simulink library "platooning_custom_blocks"  (R2018b)
settings: Solver=VariableStepAuto  StartTime=0.0  StopTime=10.0  RelTol=1e-3
undefined symbols (not defined in the file): AccPdl_pdlbpt, AccPdl_spdbpt, AccPdl_trqMap, adj_motEffMap, BETModel, BrkPdl_brkTrq, BrkPdl_pdlbpt, Cd_Map, Cd_Map_T2, CT_accPdl_pdlbpt, CT_accPdl_spdbpt, CT_accPdl_trqMap, CT_brkPdl_brkTrq, CT_brkPdl_pdlbpt, CTModel, d_11, d_22, DiscIntNeverNeededParam, init_veh_spd_mps, max_Cd_frac, min_Cd_frac, motSpdVec, motTrqVec, msk_init_pos_m, msk_mot_cont_trq, msk_mot_num, msk_mot_spd_bpt, N_OptResults, sim_t_step, simDrv, SPHETModel, t_step
libraries: simulink x19, $bdroot x16, dspstat3 x2, custom_func x1
(part 2 of 5)

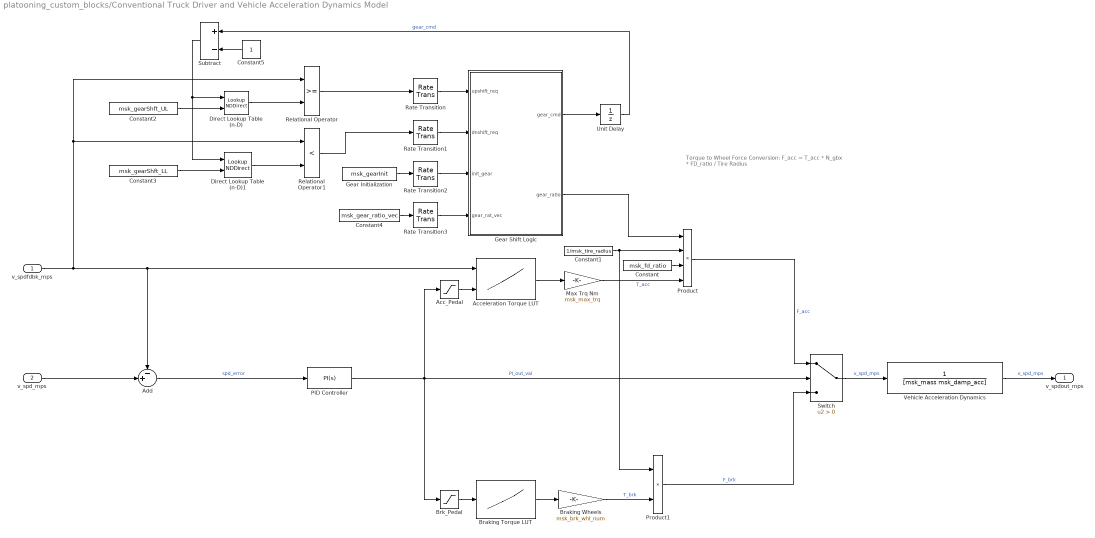
== system platooning_custom_blocks/Conventional Truck Driver and Vehicle Acceleration Dynamics Model ==
  note: Torque to Wheel Force Conversion:
      | F_acc = T_acc * N_gbx * FD_ratio / Tire Radius
  v_spdfdbk_mps : Inport
  v_spd_mps : Inport  Port=2
  Acc_Pedal : Saturate  UpperLimit=1  LowerLimit=0
  Acceleration Torque LUT : Lookup_n-D  BreakpointsForDimension1=msk_acc_spdbpt  BreakpointsForDimension2=msk_acc_pdlbpt  Table=msk_acc_trqmap  InternalRulePriority=Speed  RndMeth=Simplest  InputSameDT=on
  Add : Sum  Inputs=-+|
  Braking Torque LUT : Lookup_n-D  NumberOfTableDimensions=1  BreakpointsForDimension1=msk_brk_pdlbpt  Table=msk_brk_trq  InternalRulePriority=Speed  RndMeth=Simplest  InputSameDT=on
  Braking Wheels : Gain  Gain=msk_brk_whl_num
  Brk_Pedal : Saturate  UpperLimit=0  LowerLimit=-1
  Constant : Constant  Value=msk_fd_ratio
  Constant1 : Constant  Value=1/msk_tire_radius
  Constant2 : Constant  Value=msk_gearShft_UL
  Constant3 : Constant  Value=msk_gearShft_LL
  Constant4 : Constant  Value=msk_gear_ratio_vec
  Constant5 : Constant
  Direct Lookup Table (n-D) : LookupNDDirect  NumberOfTableDimensions=1  TableIsInput=on
  Direct Lookup Table (n-D)1 : LookupNDDirect  NumberOfTableDimensions=1  TableIsInput=on
  Gear Initialization : Constant  Value=msk_gearInit
  Gear Shift Logic : MATLAB Function  TreatAsAtomicUnit=on
  Max Trq Nm : Gain  Gain=msk_max_trq
  PID Controller : simulink/Continuous/PID Controller  Controller=PI  Form=Parallel  TimeDomain=Continuous-time  SampleTime=-1  IntegratorMethod=Forward Euler  FilterMethod=Forward Euler  ControllerParametersSource=internal  P=msk_Kp  I=msk_Ki  D=0  UseFilter=on  N=100  TunerSelectOption=Transfer Function Based (PID Tuner App)  InitialConditionSource=internal  InitialConditionForIntegrator=0  InitialConditionForFilter=0  DifferentiatorICPrevScaledInput=0  ExternalReset=none  TrackingMode=off  Kt=1  LimitOutput=on  UpperSaturationLimit=1  LowerSaturationLimit=-1  LinearizeAsGain=on  AntiWindupMode=clamping  Kb=1  POutMin=[]  POutMax=[]  IOutMin=[]  IOutMax=[]  DOutMin=[]  DOutMax=[]  NOutMin=[]  NOutMax=[]  SumOutMin=[]  SumOutMax=[]  SaturationOutMin=[]  SaturationOutMax=[]  PParamMin=[]  PParamMax=[]  IParamMin=[]  IParamMax=[]  DParamMin=[]  DParamMax=[]  NParamMin=[]  NParamMax=[]  KbParamMin=[]  KbParamMax=[]  KtParamMin=[]  KtParamMax=[]  KbOutMin=[]  KbOutMax=[]  KtOutMin=[]  KtOutMax=[]  IntegratorOutMin=[]  IntegratorOutMax=[]  FilterOutMin=[]  FilterOutMax=[]  SumI1OutMin=[]  SumI1OutMax=[]  SumI2OutMin=[]  SumI2OutMax=[]  SumI3OutMin=[]  SumI3OutMax=[]  SumI4OutMin=[]  SumI4OutMax=[]  SumDOutMin=[]  SumDOutMax=[]  DifferentiatorOutMin=[]  DifferentiatorOutMax=[]  FilterDiffOutCoefMin=[]  FilterDiffOutCoefMax=[]  ReciprocalOutMin=[]  ReciprocalOutMax=[]  SumDenOutMin=[]  SumDenOutMax=[]  SumNumOutMin=[]  SumNumOutMax=[]  DivideOutMin=[]  DivideOutMax=[]  IntegratorContinuousStateAttributes=''  IntegratorStateMustResolveToSignalObject=off  IntegratorRTWStateStorageClass=Auto  FilterContinuousStateAttributes=''  FilterStateMustResolveToSignalObject=off  FilterRTWStateStorageClass=Auto  ParallelPVariant=InternalParameters  IdealPVariant=Disabled  IVariant=InternalParameters  DVariant=Disabled  IntegratorVariant=Continuous  SatVariant=Enabled  AWVariant=ContClampingParallel  PCopyVariant=Disabled  TRVariant=Disabled  FdbkBlocksVariant=Forward  IdealPFdbkVariant=Disabled  SatFdbkVariant=Disabled  DerivativeFilterVariant=Disabled  NVariant=Disabled  NCopyVariant=Disabled_SignalSpec  FilterICVariant=Disabled  IntegratorICVariant=InternalICs  ExternalResetVariant=Disabled  TRSumVariant=Passthrough  SumFdbkVariant=Disabled  SumVariant=Sum_PI
  Product : Product  Inputs=4
  Product1 : Product
  Rate Transition{,1..3} (4 alike) : RateTransition  OutPortSampleTime=msk_t_step
  Relational Operator : RelationalOperator  OutDataTypeStr=boolean  RndMeth=Simplest
  Relational Operator1 : RelationalOperator  Operator=<  OutDataTypeStr=boolean  RndMeth=Simplest
  Subtract : Sum  Inputs=+-
  Switch : Switch  Criteria=u2 > Threshold
  Unit Delay : UnitDelay  SampleTime=-1
  Vehicle Acceleration Dynamics : TransferFcn  Denominator=[msk_mass msk_damp_acc]
  v_spdout_mps : Outport
  wires:
  Switch/1 -> Vehicle Acceleration Dynamics/1  "v_spd_mps"
  Vehicle Acceleration Dynamics/1 -> v_spdout_mps/1  "v_spd_mps"
  Braking Wheels/1 -> Product1/2  "T_brk"
  Max Trq Nm/1 -> Product/4  "T_acc"
  Rate Transition3/1 -> Gear Shift Logic/4(gear_rat_vec)
  Rate Transition2/1 -> Gear Shift Logic/3(init_gear)
  Rate Transition1/1 -> Gear Shift Logic/2(dnshift_req)
  Rate Transition/1 -> Gear Shift Logic/1(upshift_req)
  Braking Torque LUT/1 -> Braking Wheels/1
  PID Controller/1 -> Switch/2, Brk_Pedal/1, Acc_Pedal/1  "PI_out_val"
  Acceleration Torque LUT/1 -> Max Trq Nm/1
  v_spdfdbk_mps/1 -> Relational Operator1/1, Relational Operator/1, Add/1, Acceleration Torque LUT/1
  v_spd_mps/1 -> Add/2
  Product1/1 -> Switch/3  "F_brk"
  Product/1 -> Switch/1  "F_acc"
  Add/1 -> PID Controller/1  "spd_error"
  Acc_Pedal/1 -> Acceleration Torque LUT/2
  Brk_Pedal/1 -> Braking Torque LUT/1
  Constant/1 -> Product/3
  Constant1/1 -> Product1/1, Product/2
  Direct Lookup Table (n-D)/1 -> Relational Operator/2
  Constant2/1 -> Direct Lookup Table (n-D)/2
  Constant3/1 -> Direct Lookup Table (n-D)1/2
  Direct Lookup Table (n-D)1/1 -> Relational Operator1/2
  Relational Operator/1 -> Rate Transition/1
  Relational Operator1/1 -> Rate Transition1/1
  Gear Initialization/1 -> Rate Transition2/1
  Gear Shift Logic/1(gear_cmd) -> Unit Delay/1
  Gear Shift Logic/2(gear_ratio) -> Product/1
  Constant4/1 -> Rate Transition3/1
  Unit Delay/1 -> Subtract/1  "gear_cmd"
  Constant5/1 -> Subtract/2
  Subtract/1 -> Direct Lookup Table (n-D)1/1, Direct Lookup Table (n-D)/1

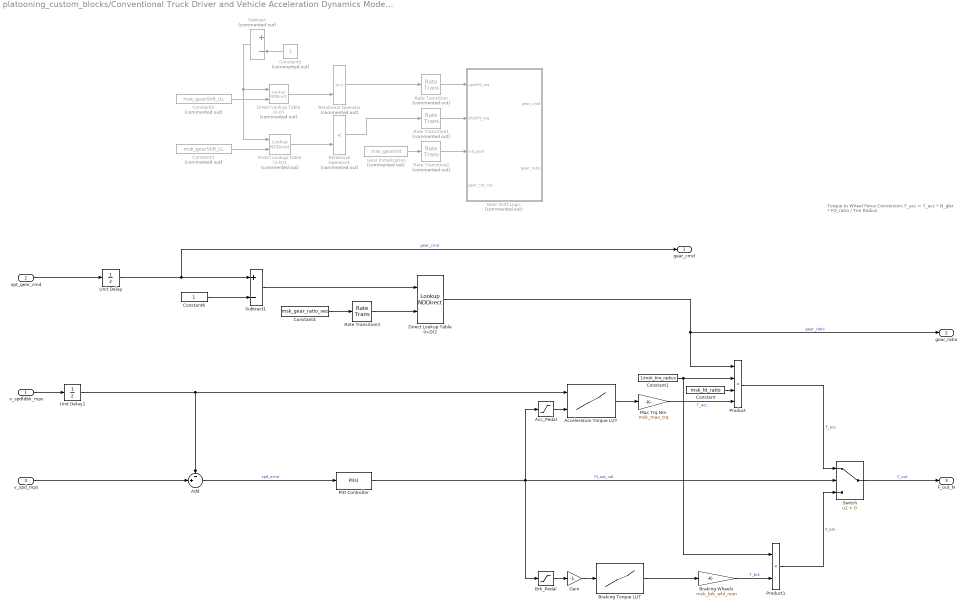
== system platooning_custom_blocks/Conventional Truck Driver and Vehicle Acceleration Dynamics Model - Force Output ==
  note: Torque to Wheel Force Conversion:
      | F_acc = T_acc * N_gbx * FD_ratio / Tire Radius
  v_spdfdbk_mps : Inport
  opt_gear_cmd : Inport  Port=2
  v_spd_mps : Inport  Port=3
  Acc_Pedal : Saturate  UpperLimit=1  LowerLimit=0
  Acceleration Torque LUT : Lookup_n-D  BreakpointsForDimension1=msk_acc_spdbpt  BreakpointsForDimension2=msk_acc_pdlbpt  Table=msk_acc_trqmap  InternalRulePriority=Speed  RndMeth=Simplest  InputSameDT=on
  Add : Sum  Inputs=-+|
  Braking Torque LUT : Lookup_n-D  NumberOfTableDimensions=1  BreakpointsForDimension1=msk_brk_pdlbpt  Table=msk_brk_trq * -1  InternalRulePriority=Speed  RndMeth=Simplest  InputSameDT=on
  Braking Wheels : Gain  Gain=msk_brk_whl_num
  Brk_Pedal : Saturate  UpperLimit=0  LowerLimit=-1
  Constant : Constant  Value=msk_fd_ratio
  Constant1 : Constant  Value=1/msk_tire_radius
  Constant2 : Constant  Commented=on  Value=msk_gearShft_UL
  Constant3 : Constant  Commented=on  Value=msk_gearShft_LL
  Constant4 : Constant  Value=msk_gear_ratio_vec
  Constant5 : Constant  Commented=on
  Constant6 : Constant
  Direct Lookup Table (n-D) : LookupNDDirect  Commented=on  NumberOfTableDimensions=1  TableIsInput=on
  Direct Lookup Table (n-D)1 : LookupNDDirect  Commented=on  NumberOfTableDimensions=1  TableIsInput=on
  Direct Lookup Table (n-D)2 : LookupNDDirect  NumberOfTableDimensions=1  TableIsInput=on
  Gain : Gain  Gain=-1
  Gear Initialization : Constant  Commented=on  Value=msk_gearInit
  Gear Shift Logic : MATLAB Function  Commented=on  TreatAsAtomicUnit=on
  Max Trq Nm : Gain  Gain=msk_max_trq
  PID Controller : simulink/Continuous/PID Controller  Controller=PI  Form=Parallel  TimeDomain=Continuous-time  SampleTime=-1  IntegratorMethod=Forward Euler  FilterMethod=Forward Euler  ControllerParametersSource=internal  P=msk_Kp  I=msk_Ki  D=0  UseFilter=on  N=100  TunerSelectOption=Transfer Function Based (PID Tuner App)  InitialConditionSource=internal  InitialConditionForIntegrator=0  InitialConditionForFilter=0  DifferentiatorICPrevScaledInput=0  ExternalReset=none  TrackingMode=off  Kt=1  LimitOutput=on  UpperSaturationLimit=1  LowerSaturationLimit=-1  LinearizeAsGain=on  AntiWindupMode=clamping  Kb=1  POutMin=[]  POutMax=[]  IOutMin=[]  IOutMax=[]  DOutMin=[]  DOutMax=[]  NOutMin=[]  NOutMax=[]  SumOutMin=[]  SumOutMax=[]  SaturationOutMin=[]  SaturationOutMax=[]  PParamMin=[]  PParamMax=[]  IParamMin=[]  IParamMax=[]  DParamMin=[]  DParamMax=[]  NParamMin=[]  NParamMax=[]  KbParamMin=[]  KbParamMax=[]  KtParamMin=[]  KtParamMax=[]  KbOutMin=[]  KbOutMax=[]  KtOutMin=[]  KtOutMax=[]  IntegratorOutMin=[]  IntegratorOutMax=[]  FilterOutMin=[]  FilterOutMax=[]  SumI1OutMin=[]  SumI1OutMax=[]  SumI2OutMin=[]  SumI2OutMax=[]  SumI3OutMin=[]  SumI3OutMax=[]  SumI4OutMin=[]  SumI4OutMax=[]  SumDOutMin=[]  SumDOutMax=[]  DifferentiatorOutMin=[]  DifferentiatorOutMax=[]  FilterDiffOutCoefMin=[]  FilterDiffOutCoefMax=[]  ReciprocalOutMin=[]  ReciprocalOutMax=[]  SumDenOutMin=[]  SumDenOutMax=[]  SumNumOutMin=[]  SumNumOutMax=[]  DivideOutMin=[]  DivideOutMax=[]  IntegratorContinuousStateAttributes=''  IntegratorStateMustResolveToSignalObject=off  IntegratorRTWStateStorageClass=Auto  FilterContinuousStateAttributes=''  FilterStateMustResolveToSignalObject=off  FilterRTWStateStorageClass=Auto  ParallelPVariant=InternalParameters  IdealPVariant=Disabled  IVariant=InternalParameters  DVariant=Disabled  IntegratorVariant=Continuous  SatVariant=Enabled  AWVariant=ContClampingParallel  PCopyVariant=Disabled  TRVariant=Disabled  FdbkBlocksVariant=Forward  IdealPFdbkVariant=Disabled  SatFdbkVariant=Disabled  DerivativeFilterVariant=Disabled  NVariant=Disabled  NCopyVariant=Disabled_SignalSpec  FilterICVariant=Disabled  IntegratorICVariant=InternalICs  ExternalResetVariant=Disabled  TRSumVariant=Passthrough  SumFdbkVariant=Disabled  SumVariant=Sum_PI
  Product : Product  Inputs=4
  Product1 : Product
  Rate Transition : RateTransition  Commented=on  OutPortSampleTime=msk_t_step
  Rate Transition1 : RateTransition  Commented=on  OutPortSampleTime=msk_t_step
  Rate Transition2 : RateTransition  Commented=on  OutPortSampleTime=msk_t_step
  Rate Transition3 : RateTransition  OutPortSampleTime=msk_t_step
  Relational Operator : RelationalOperator  Commented=on  OutDataTypeStr=boolean  RndMeth=Simplest
  Relational Operator1 : RelationalOperator  Commented=on  Operator=<  OutDataTypeStr=boolean  RndMeth=Simplest
  Subtract : Sum  Commented=on  Inputs=+-
  Subtract1 : Sum  Inputs=+-
  Switch : Switch  Criteria=u2 > Threshold
  Unit Delay : UnitDelay  InitialCondition=msk_gearInit  SampleTime=-1
  Unit Delay1 : UnitDelay  SampleTime=-1
  gear_cmd : Outport
  gear_ratio : Outport  Port=2
  F_out_N : Outport  Port=3
  wires:
  Gain/1 -> Braking Torque LUT/1
  Unit Delay1/1 -> Acceleration Torque LUT/1, Add/1
  Switch/1 -> F_out_N/1  "F_out"
  Braking Wheels/1 -> Product1/2  "T_brk"
  Max Trq Nm/1 -> Product/4  "T_acc"
  Rate Transition2/1 -> Gear Shift Logic/3(init_gear)
  Rate Transition1/1 -> Gear Shift Logic/2(dnshift_req)
  Rate Transition/1 -> Gear Shift Logic/1(upshift_req)
  Braking Torque LUT/1 -> Braking Wheels/1
  PID Controller/1 -> Switch/2, Brk_Pedal/1, Acc_Pedal/1  "PI_out_val"
  Acceleration Torque LUT/1 -> Max Trq Nm/1
  v_spdfdbk_mps/1 -> Unit Delay1/1
  v_spd_mps/1 -> Add/2
  Product1/1 -> Switch/3  "F_brk"
  Product/1 -> Switch/1  "F_acc"
  Add/1 -> PID Controller/1  "spd_error"
  Acc_Pedal/1 -> Acceleration Torque LUT/2
  Brk_Pedal/1 -> Gain/1
  Constant/1 -> Product/3
  Constant1/1 -> Product1/1, Product/2
  Direct Lookup Table (n-D)/1 -> Relational Operator/2
  Constant2/1 -> Direct Lookup Table (n-D)/2
  Constant3/1 -> Direct Lookup Table (n-D)1/2
  Direct Lookup Table (n-D)1/1 -> Relational Operator1/2
  Relational Operator/1 -> Rate Transition/1
  Relational Operator1/1 -> Rate Transition1/1
  Gear Initialization/1 -> Rate Transition2/1
  Direct Lookup Table (n-D)2/1 -> Product/1, gear_ratio/1  "gear_ratio"
  Constant4/1 -> Rate Transition3/1
  Unit Delay/1 -> gear_cmd/1, Subtract1/1  "gear_cmd"
  Constant5/1 -> Subtract/2
  Subtract/1 -> Direct Lookup Table (n-D)1/1, Direct Lookup Table (n-D)/1
  Rate Transition3/1 -> Direct Lookup Table (n-D)2/2
  opt_gear_cmd/1 -> Unit Delay/1
  Subtract1/1 -> Direct Lookup Table (n-D)2/1
  Constant6/1 -> Subtract1/2

== system platooning_custom_blocks/Lead Truck Powertrain Variant Subsystem ==
  note: 1) Add Subsystem or Model blocks as valid variant choices.
      | 2) You cannot connect blocks at this level. At simulation, connectivity is automatically
      | determined, based on the active variant and port name matching.
  From_DTIL_BUS : Inport
  V_SPD : Inport  Port=2
  F_Dist_m : Inport  Port=3
  Cd : Inport  Port=4
  From_PCL : Inport  Port=5
  Init_Pos_m : Inport  Port=6
  Battery Electric Truck : $bdroot/Battery Electric Truck  SystemSampleTime=-1  VariantControl=LT.Type == 3
  Conventional Truck : $bdroot/Conventional Truck  SystemSampleTime=-1  VariantControl=LT.Type == 1
  Series Parallel Hybrid Electric Truck : $bdroot/Series Parallel Hybrid Electric Truck  SystemSampleTime=-1  VariantControl=LT.Type == 2
  To_PCL : Outport

== system platooning_custom_blocks/Mid Truck Powertrain Variant Subsystem ==
  note: 1) Add Subsystem or Model blocks as valid variant choices.
      | 2) You cannot connect blocks at this level. At simulation, connectivity is automatically
      | determined, based on the active variant and port name matching.
  From_DTIL_BUS : Inport
  V_SPD : Inport  Port=2
  F_Dist_m : Inport  Port=3
  Cd : Inport  Port=4
  From_PCL : Inport  Port=5
  Init_Pos_m : Inport  Port=6
  Battery Electric Truck : $bdroot/Battery Electric Truck  SystemSampleTime=-1  VariantControl=MT.Type == 3
  Conventional Truck : $bdroot/Conventional Truck  SystemSampleTime=-1  VariantControl=MT.Type == 1
  Series Parallel Hybrid Electric Truck : $bdroot/Series Parallel Hybrid Electric Truck  SystemSampleTime=-1  VariantControl=MT.Type == 2
  To_PCL : Outport

== system platooning_custom_blocks/Optimal Gear Shift Algorithm ==
  P_dem_W : Inport
  veh_spd_mps : Inport  Port=2
  Bus Creator : BusCreator  Inputs=10
  Constant : Constant  Value=eps
  Divide : Product  Inputs=*/
  Fuel LUT @ Gear 1 : Lookup_n-D  BreakpointsForDimension1=CTModel.eng_map_trq_bpt(10:end) * (CTModel.gear_ratios(1) * CTModel.fd_ratio)  BreakpointsForDimension2=(CTModel.eng_map_spd_bpt * 0.1047 * CTModel.ld_tire_rad_m)/(CTModel.gear_ratios(1) * CTModel.fd_ratio)  Table=CTModel.eng_fuel_map(10:end,:)  ExtrapMethod=Clip  UseLastTableValue=on  InternalRulePriority=Speed  RndMeth=Simplest  InputSameDT=on
  Fuel LUT @ Gear 10 : Lookup_n-D  BreakpointsForDimension1=CTModel.eng_map_trq_bpt(10:end) * (CTModel.gear_ratios(10) * CTModel.fd_ratio)  BreakpointsForDimension2=(CTModel.eng_map_spd_bpt * 0.1047 * CTModel.ld_tire_rad_m)/(CTModel.gear_ratios(10) * CTModel.fd_ratio)  Table=CTModel.eng_fuel_map(10:end,:)  ExtrapMethod=Clip  UseLastTableValue=on  InternalRulePriority=Speed  RndMeth=Simplest  InputSameDT=on
  Fuel LUT @ Gear 2 : Lookup_n-D  BreakpointsForDimension1=CTModel.eng_map_trq_bpt(10:end) * (CTModel.gear_ratios(2) * CTModel.fd_ratio)  BreakpointsForDimension2=(CTModel.eng_map_spd_bpt * 0.1047 * CTModel.ld_tire_rad_m)/(CTModel.gear_ratios(2) * CTModel.fd_ratio)  Table=CTModel.eng_fuel_map(10:end,:)  ExtrapMethod=Clip  UseLastTableValue=on  InternalRulePriority=Speed  RndMeth=Simplest  InputSameDT=on
  Fuel LUT @ Gear 3 : Lookup_n-D  BreakpointsForDimension1=CTModel.eng_map_trq_bpt(10:end) * (CTModel.gear_ratios(3) * CTModel.fd_ratio)  BreakpointsForDimension2=(CTModel.eng_map_spd_bpt * 0.1047 * CTModel.ld_tire_rad_m)/(CTModel.gear_ratios(3) * CTModel.fd_ratio)  Table=CTModel.eng_fuel_map(10:end,:)  ExtrapMethod=Clip  UseLastTableValue=on  InternalRulePriority=Speed  RndMeth=Simplest  InputSameDT=on
  Fuel LUT @ Gear 4 : Lookup_n-D  BreakpointsForDimension1=CTModel.eng_map_trq_bpt(10:end) * (CTModel.gear_ratios(4) * CTModel.fd_ratio)  BreakpointsForDimension2=(CTModel.eng_map_spd_bpt * 0.1047 * CTModel.ld_tire_rad_m)/(CTModel.gear_ratios(4) * CTModel.fd_ratio)  Table=CTModel.eng_fuel_map(10:end,:)  ExtrapMethod=Clip  UseLastTableValue=on  InternalRulePriority=Speed  RndMeth=Simplest  InputSameDT=on
  Fuel LUT @ Gear 5 : Lookup_n-D  BreakpointsForDimension1=CTModel.eng_map_trq_bpt(10:end) * (CTModel.gear_ratios(5) * CTModel.fd_ratio)  BreakpointsForDimension2=(CTModel.eng_map_spd_bpt * 0.1047 * CTModel.ld_tire_rad_m)/(CTModel.gear_ratios(5) * CTModel.fd_ratio)  Table=CTModel.eng_fuel_map(10:end,:)  ExtrapMethod=Clip  UseLastTableValue=on  InternalRulePriority=Speed  RndMeth=Simplest  InputSameDT=on
  Fuel LUT @ Gear 6 : Lookup_n-D  BreakpointsForDimension1=CTModel.eng_map_trq_bpt(10:end) * (CTModel.gear_ratios(6) * CTModel.fd_ratio)  BreakpointsForDimension2=(CTModel.eng_map_spd_bpt * 0.1047 * CTModel.ld_tire_rad_m)/(CTModel.gear_ratios(6) * CTModel.fd_ratio)  Table=CTModel.eng_fuel_map(10:end,:)  ExtrapMethod=Clip  UseLastTableValue=on  InternalRulePriority=Speed  RndMeth=Simplest  InputSameDT=on
  Fuel LUT @ Gear 7 : Lookup_n-D  BreakpointsForDimension1=CTModel.eng_map_trq_bpt(10:end) * (CTModel.gear_ratios(7) * CTModel.fd_ratio)  BreakpointsForDimension2=(CTModel.eng_map_spd_bpt * 0.1047 * CTModel.ld_tire_rad_m)/(CTModel.gear_ratios(7) * CTModel.fd_ratio)  Table=CTModel.eng_fuel_map(10:end,:)  ExtrapMethod=Clip  UseLastTableValue=on  InternalRulePriority=Speed  RndMeth=Simplest  InputSameDT=on
  Fuel LUT @ Gear 8 : Lookup_n-D  BreakpointsForDimension1=CTModel.eng_map_trq_bpt(10:end) * (CTModel.gear_ratios(8) * CTModel.fd_ratio)  BreakpointsForDimension2=(CTModel.eng_map_spd_bpt * 0.1047 * CTModel.ld_tire_rad_m)/(CTModel.gear_ratios(8) * CTModel.fd_ratio)  Table=CTModel.eng_fuel_map(10:end,:)  ExtrapMethod=Clip  UseLastTableValue=on  InternalRulePriority=Speed  RndMeth=Simplest  InputSameDT=on
  Fuel LUT @ Gear 9 : Lookup_n-D  BreakpointsForDimension1=CTModel.eng_map_trq_bpt(10:end) * (CTModel.gear_ratios(9) * CTModel.fd_ratio)  BreakpointsForDimension2=(CTModel.eng_map_spd_bpt * 0.1047 * CTModel.ld_tire_rad_m)/(CTModel.gear_ratios(9) * CTModel.fd_ratio)  Table=CTModel.eng_fuel_map(10:end,:)  ExtrapMethod=Clip  UseLastTableValue=on  InternalRulePriority=Speed  RndMeth=Simplest  InputSameDT=on
  Loaded Tire Radius m : Gain  Gain=msk_tire_radius_m
  Minimum Function : MATLAB Function  TreatAsAtomicUnit=on
  Switch : Switch  Criteria=u2 > Threshold
  Transmission Efficiency : Gain  Gain=1/msk_trns_eff_avg
  init_gear : Constant  Value=msk_init_gear
  opt_gear : Outport
  wires:
  Fuel LUT @ Gear 4/1 -> Bus Creator/4  "m_fuel_Gear_4"
  Loaded Tire Radius m/1 -> Transmission Efficiency/1
  init_gear/1 -> Minimum Function/2(prev_gear)
  veh_spd_mps/1 -> Switch/2, Switch/1, Fuel LUT @ Gear 1/2, Fuel LUT @ Gear 10/2, Fuel LUT @ Gear 9/2, Fuel LUT @ Gear 8/2, Fuel LUT @ Gear 7/2, Fuel LUT @ Gear 6/2, Fuel LUT @ Gear 5/2, Fuel LUT @ Gear 4/2, Fuel LUT @ Gear 3/2, Fuel LUT @ Gear 2/2
  Constant/1 -> Switch/3
  Fuel LUT @ Gear 1/1 -> Bus Creator/1  "m_fuel_Gear_1"
  Fuel LUT @ Gear 7/1 -> Bus Creator/7  "m_fuel_Gear_7"
  Minimum Function/1(opt_gear) -> opt_gear/1
  Fuel LUT @ Gear 10/1 -> Bus Creator/10  "m_fuel_Gear_10"
  Switch/1 -> Divide/2
  Fuel LUT @ Gear 3/1 -> Bus Creator/3  "m_fuel_Gear_3"
  Divide/1 -> Fuel LUT @ Gear 10/1, Fuel LUT @ Gear 9/1, Fuel LUT @ Gear 8/1, Fuel LUT @ Gear 7/1, Fuel LUT @ Gear 6/1, Fuel LUT @ Gear 5/1, Fuel LUT @ Gear 4/1, Fuel LUT @ Gear 3/1, Fuel LUT @ Gear 2/1, Fuel LUT @ Gear 1/1
  Fuel LUT @ Gear 9/1 -> Bus Creator/9  "m_fuel_Gear_9"
  Fuel LUT @ Gear 8/1 -> Bus Creator/8  "m_fuel_Gear_8"
  Fuel LUT @ Gear 2/1 -> Bus Creator/2  "m_fuel_Gear_2"
  Bus Creator/1 -> Minimum Function/1(m_fuel_vec)  "m_fuel_opt_bus"
  Fuel LUT @ Gear 6/1 -> Bus Creator/6  "m_fuel_Gear_6"
  Fuel LUT @ Gear 5/1 -> Bus Creator/5  "m_fuel_Gear_5"
  P_dem_W/1 -> Loaded Tire Radius m/1
  Transmission Efficiency/1 -> Divide/1

== system platooning_custom_blocks/Platoon Cd Map ==
  LT_MT_Dist : Inport
  MT_TT_Dist : Inport  Port=2
  Constant : Constant  Value=pos
  Constant1 : Constant  Value=max_Cd_frac * msk_cd_avg
  Constant2 : Constant  Value=min_Cd_frac * msk_cd_avg
  Constant3 : Constant  Value=msk_platoon_type
  Constant4 : Constant  Value=msk_cd_avg
  MATLAB Function : MATLAB Function  TreatAsAtomicUnit=on
  Multiport Switch : MultiPortSwitch
  Platoon Cd Map - 2 Truck : Lookup_n-D  BreakpointsForDimension1=msk_d1_bpt  BreakpointsForDimension2=[1:2]  Table=msk_platoon_cd_map_t2  InternalRulePriority=Speed  RndMeth=Simplest  InputSameDT=on
  Platoon Cd Map - 3 Truck : Lookup_n-D  NumberOfTableDimensions=3  BreakpointsForDimension1=msk_d1_bpt  BreakpointsForDimension2=msk_d2_bpt  BreakpointsForDimension3=[1,2,3]  Table=msk_platoon_cd_map  InternalRulePriority=Speed  RndMeth=Simplest  InputSameDT=on
  Cd : Outport
  wires:
  Constant4/1 -> Multiport Switch/2
  Constant3/1 -> Multiport Switch/1
  Platoon Cd Map - 2 Truck/1 -> Multiport Switch/3
  Platoon Cd Map - 3 Truck/1 -> Multiport Switch/4
  Constant2/1 -> MATLAB Function/3(Cd_min)
  Constant1/1 -> MATLAB Function/2(Cd_max)
  Multiport Switch/1 -> MATLAB Function/1(Cd_input)
  MT_TT_Dist/1 -> Platoon Cd Map - 3 Truck/2
  LT_MT_Dist/1 -> Platoon Cd Map - 3 Truck/1, Platoon Cd Map - 2 Truck/1
  Constant/1 -> Platoon Cd Map - 3 Truck/3, Platoon Cd Map - 2 Truck/2
  MATLAB Function/1(Cd_output) -> Cd/1

== system platooning_custom_blocks/Series Parallel Hybrid Electric Truck ==
  From_DTIL_BUS : Inport
  V_SPD : Inport  Port=2
  F_Dist_m : Inport  Port=3
  Cd : Inport  Port=4
  From_PCL : Inport  Port=5
  Init_Pos_m : Inport  Port=6
  2 DOF Longitudinal Dynamics Model - Force Input : $bdroot/2 DOF Longitudinal Dynamics Model - Force Input  msk_mass=SPHETModel.veh_mass_kg  msk_Af=SPHETModel.Af_m2  msk_Cd=SPHETModel.Cd_avg * ones([3 1])  msk_Cd_bpt=[5;10;15]  msk_r_tire=SPHETModel.ld_tire_rad_m  msk_v_init=init_veh_spd_mps  msk_roadType=Smooth Concrete  msk_rho_air=1.227  msk_tstep=sim_t_step
  Bus Creator : BusCreator  Inputs=3
  Bus Creator1 : BusCreator  Inputs=4
  Bus Creator2 : BusCreator  Inputs=4
  Bus Creator3 : BusCreator  Inputs=4
  Bus Selector : BusSelector  OutputSignals=opt_gear
  Bus Selector1 : BusSelector  OutputSignals=EC_BUS.blndElecEC_Wh_m,State_BUS.DistTrvld_m
  Bus Selector2 : BusSelector  OutputSignals=tail_grade_pct
  Bus Selector3 : BusSelector  OutputSignals=clock
  Series Parallel Hybrid Electric Post-Processing : Subsystem  mask{msk_cell_Q_Ah=SPHETModel.Q_cell_max_Ah, msk_cell_Vnom=SPHETModel.V_cell_nom, msk_batt_Ns=SPHETModel.Ns, msk_batt_Np=SPHETModel.Np, msk_batt_Nmod=SPHETModel.Nmod, msk_batt_soc_init=0.8, msk_fuel_init_liters=SPHETModel.fuelTankCap_L, msk_fuel_rho_kgpl=SPHETModel.fuelrho_kgpl, msk_fuel_lhv_kwhpkg=SPHETModel.fuelLHV_kwhpkg, msk_distwin=1000}
      mask prompts: msk_cell_Q_Ah "Battery cell capacity, Q [Ah]:"; msk_cell_Vnom "Battery cell nominal voltage, Vnom [V]:"; msk_batt_Ns "Number of cells in series, Ns [-]:"; msk_batt_Np "Number of cells in parallel, Np [-]:"; msk_batt_Nmod "Number of modules, Nmod [-]:"; msk_batt_soc_init "Battery initial SOC, SOCinit/100 :"; msk_fuel_init_liters "Initial fuel capacity [US gallons]:"; msk_fuel_rho_kgpl "Fuel density [kg/L]:"; msk_fuel_lhv_kwhpkg "Fuel LHV [kWh/kg]:"; msk_distwin "Short term averaging, distance window [m]:"
      mask DialogControl DescGroupVar Prompt: Post-Processing Block - Battery Electric Vehicle
      mask DialogControl DescTextVar Prompt: This block computes overall energy consumption and distance-to-empty for a battery electric vehicle.
      mask DialogControl ParameterGroupVar Prompt: Battery Parameters
      mask DialogControl Container3 Prompt: Fuel Parameters
      mask DialogControl Container4 Prompt: Averaging Parameters
  Series Parallel Hybrid Electric Powertrain Power Loss Model : Subsystem  mask{msk_eng_pk_trq_vec=SPHETModel.peak_eng_trq_map, msk_eng_pk_mtr_trq=SPHETModel.mtr_eng_trq_map, msk_eng_trq_spd_bpt=SPHETModel.peak_eng_trq_spd_bpt, msk_eng_fuel_map=SPHETModel.eng_fuel_map, msk_eng_trq_bpt=SPHETModel.eng_map_trq_bpt, msk_eng_spd_bpt=SPHETModel.eng_map_spd_bpt, msk_fuel_init_liters=SPHETModel.fuelTankCap_L, msk_rho_fuel_kgpL=SPHETModel.fuelrho_kgpl, msk_gen_ctl_Kp=0.1, msk_gen_ctl_Ki=0.001, msk_gen_mtr_cont_trq=SPHETModel.cont_gen_mtr_trq_map, msk_gen_mtr_eff_map=SPHETModel.gen_mtr_eff_map, msk_gen_mtr_trqbpt=SPHETModel.gen_mtr_trqbpt, msk_gen_mtr_spdbpt=SPHETModel.gen_mtr_spdbpt, msk_mot_eff=SPHETModel.mtr_eff, msk_gear_ratio_vec=SPHETModel.gear_ratios, msk_gear_eff_vec=SPHETModel.gear_eff, msk_fd_ratio=SPHETModel.fd_ratio, msk_drv_eff=0.98, msk_plnt_m_r_ratio=SPHETModel.mg_ratio_mot_out, msk_plnt_c_r_ratio=SPHETModel.mg_ratio_eng_out, msk_plnt_s_r_ratio=1/SPHETModel.mg_ratio_out_gen, msk_plnt_c_s_ratio=SPHETModel.mg_ratio_eng_gen, msk_plnt_gear_eff=SPHETModel.plnt_gear_eff, msk_tire_radius_m=SPHETModel.ld_tire_rad_m, msk_cell_Q_Ah=SPHETModel.Q_cell_max_Ah, msk_cell_Vnom=SPHETModel.V_cell_nom, msk_batt_Ns=SPHETModel.Ns, msk_batt_Np=SPHETModel.Np, msk_batt_Nmod=SPHETModel.Nmod, msk_batt_soc_init=0.8, msk_dchglim10s=SPHETModel.DchgCurrLim_10sAvg_A, msk_cellTempbpt=SPHETModel.cellTempbpt_C, msk_soc_bpt=SPHETModel.socbpt, msk_batt_R0=SPHETModel.batt_R0, msk_batt_R1=SPHETModel.batt_R1, msk_batt_R2=SPHETModel.batt_R2, msk_batt_C1=SPHETModel.batt_C1, msk_batt_C2=SPHETModel.batt_C2, msk_batt_soc_bpt=SPHETModel.batt_socbpt, msk_P_aux_mech_load=SPHETModel.P_aux_mech, msk_P_aux_elec_load=SPHETModel.P_aux_elec, msk_P_aux_load_frac=SPHETModel.P_aux_load_frac, msk_snr_P_aux=25, msk_t_step=sim_t_step}
      mask prompts: msk_eng_pk_trq_vec "Engine peak torque vector, propulsion [] :"; msk_eng_pk_mtr_trq "Engine peak torque vector, motoring [] :"; msk_eng_trq_spd_bpt "Engine torque speed breakpoint [] :"; msk_eng_fuel_map "Engine fuel map, g/s [] :"; msk_eng_trq_bpt "Engine torque breakpoint []:"; msk_eng_spd_bpt "Engine speed breakpoint []:"; msk_fuel_init_liters "Initial fuel capacity [Liters] :"; msk_rho_fuel_kgpL "Fuel density [kg/L] :"; msk_gen_ctl_Kp "Generator load control, Proportional Gain :"; msk_gen_ctl_Ki "Generator load control, Integrator Gain :"; msk_gen_mtr_cont_trq "Generator continuous torque vector [] :"; msk_gen_mtr_eff_map "Generator motor efficiency map [] :"; msk_gen_mtr_trqbpt "Generator motor torque breakpoint [] :"; msk_gen_mtr_spdbpt "Generator speed breakpoint [] :"; msk_mot_eff "Motor efficiency/100 [-]:"; msk_gear_ratio_vec "Gear ratio vector []:"; msk_gear_eff_vec "Gear efficiency vector []:"; msk_fd_ratio "Final drive ratio :"; msk_drv_eff "Driveline efficiency :"; msk_plnt_m_r_ratio "Motor to Output ratio (M to R) :"; msk_plnt_c_r_ratio "Engine to Output ratio (C to R) :"; msk_plnt_s_r_ratio "Generator to Output ratio (S to R) :"; msk_plnt_c_s_ratio "Engine to Generator ratio (C to S) :"; msk_plnt_gear_eff "Planetary gearbox efficiency :"; msk_tire_radius_m "Loaded tire radius [m]:"; msk_cell_Q_Ah "Battery cell capacity, Q [Ah]:"; msk_cell_Vnom "Battery cell nominal voltage, Vnom [V]:"; msk_batt_Ns "Number of cells in series, Ns [-]:"; msk_batt_Np "Number of cells in parallel, Np [-]:"; msk_batt_Nmod "Number of battery modules, Nmod [-]:"; msk_batt_soc_init "Battery initial SOC [SOC/100]:"; msk_dchglim10s "Battery 10s Discharge Limit []:"; msk_cellTempbpt "Battery cell temperature breakpoint []:"; msk_soc_bpt "Battery SOC breakpoint []:"; msk_batt_R0 "Battery Resistance R0 LUT []:"; msk_batt_R1 "Battery Resistance R1 LUT []:"; msk_batt_R2 "Battery Resistance R2 LUT []:"; msk_batt_C1 "Battery Capacitance C1 LUT []:"; msk_batt_C2 "Battery Capacitance C2 LUT []:"; msk_batt_soc_bpt "Battery internal params SOC breakpoints []:"; msk_P_aux_mech_load "Auxiliary load power, mechanical [W]:"; msk_P_aux_elec_load "Auxiliary load power, electrical [W]:"; msk_P_aux_load_frac "Auxiliary load fraction [-]"; msk_snr_P_aux "Signal-to-Noise ratio [-]:"; msk_t_step "Simulation time step [s]:"
      mask DialogControl DescGroupVar Prompt: Battery Electric Powertrain Mode
      mask DialogControl DescTextVar Prompt: Parameter settings for systems and components in the Battery Electric Powertrain
      mask DialogControl Container7 Prompt: Drivetrain Parameters
      mask DialogControl Container12 Prompt: Engine Parameters
      mask DialogControl Container18 Prompt: Fuel Parameters
      mask DialogControl Container13 Prompt: Generator Parameters
      mask DialogControl Container9 Prompt: Motor Parameters
      mask DialogControl Container14 Prompt: Transmission Parameters
      mask DialogControl Container16 Prompt: P2 Hybrid Planetary Gearbox
      mask DialogControl Container15 Prompt: Vehicle Parameters
      mask DialogControl Container10 Prompt: Battery Parameters
      mask DialogControl Container4 Prompt: Internal Battery Parameters
      mask DialogControl Container11 Prompt: Auxiliary Load Parameters
      mask DialogControl Container17 Prompt: Simulation Parameters
  Series Parallel Hybrid Electric Truck Energy Management System : Subsystem  mask{msk_algoChoice=DC-ARTDP Algo, msk_regen_pwr_vec=SPHETModel.mtr_regen_pwr_vec, msk_regen_spd_bpt=SPHETModel.mtr_regen_pwr_spdbpt, msk_DistVector=simDrv.dist_mi * 1609.34, msk_OptHybMode=N_OptResults.HybModeGrp, msk_OptGenPwr=N_OptResults.optPgen_W, msk_OptMotPwr=N_OptResults.optPmot_W, msk_OptSOC=N_OptResults.optSOC_pct, msk_OptEC=N_OptResults.EC_Wh_m}
      mask prompts: msk_algoChoice "Energy Management Algorithm Choice"; msk_regen_pwr_vec "Motor regen power vector, watts []:"; msk_regen_spd_bpt "Motor regen power breakpoint - vehicle speed, mps []:"; msk_DistVector "Distance Vector:"; msk_OptHybMode "Optimal Hybrid Mode Vector:"; msk_OptGenPwr "Optimal Generator Power Vector:"; msk_OptMotPwr "Optimal Motor Power Vector:"; msk_OptSOC "Optimal SOC Vector:"; msk_OptEC "Optimal EC Vector:"
      mask init:
      | switch msk_algoChoice
      |     case 'DC-ARTDP Algo'
      |         msk_algoChoice = 1;
      |     case 'Standard SPHET Algo'
      |         msk_algoChoice = 2;
      | end
      mask TypeOptions msk_algoChoice: DC-ARTDP Algo | Standard SPHET Algo
      mask DialogControl DescGroupVar Prompt: Battery Electric Energy Management System
      mask DialogControl DescTextVar Prompt: Parameter settings for the Battery Electric Energy Management Systems
      mask DialogControl Container3 Prompt: DC-ARTDP Algorithm Parameters
  Series Parallel Hybrid Electric Truck Driver and Vehicle Acceleration Dynamics Model - Force Output : $bdroot/Series Parallel Hybrid Electric Truck Driver and  Vehicle Acceleration Dynamics Model  - Force Output  msk_mass=SPHETModel.veh_mass_kg  msk_damp_acc=800  msk_damp_brk=0.1  msk_tire_radius=SPHETModel.ld_tire_rad_m  msk_brk_whl_num=18  msk_fd_ratio=SPHETModel.fd_ratio  msk_Kp=0.1  msk_Ki=0.001  msk_t_step=sim_t_step  msk_eng_pk_trq=SPHETModel.peak_eng_trq_map  msk_eng_spd_bpt=SPHETModel.peak_eng_trq_spd_bpt  msk_gear_ratio_vec=SPHETModel.gear_ratios  msk_gearInit=1  msk_gearShft_UL=[3, 5, 9, 13, 17, 21, 25, 29, 33, 45]  msk_gearShft_LL=[0, 2, 4, 8, 12, 16, 20, 24, 28, 32]  msk_plnt_c_r_ratio=SPHETModel.mg_ratio_eng_out  msk_plnt_m_r_ratio=SPHETModel.mg_ratio_mot_out  msk_plnt_s_r_ratio=1/SPHETModel.mg_ratio_out_gen  msk_plnt_s_c_ratio=1/SPHETModel.mg_ratio_eng_gen  msk_mtr_cont_trq=SPHETModel.cont_mtr_trq_map  msk_mtr_pk_trq=SPHETModel.peak_mtr_trq_map  msk_spd_bpt=SPHETModel.cont_mtr_trq_spdbpt  msk_gear_ratio=SPHETModel.mg_ratio_mot_out  msk_num_motors=1  msk_acc_trqmap=AccPdl_trqMap  msk_acc_spdbpt=AccPdl_spdbpt  msk_acc_pdlbpt=AccPdl_pdlbpt  msk_brk_trq=BrkPdl_brkTrq  msk_brk_pdlbpt=BrkPdl_pdlbpt
  Terminator : Terminator
  Unit Delay : UnitDelay  InitialCondition=3  SampleTime=-1
  Unit Delay1 : UnitDelay  InitialCondition=3  SampleTime=-1
  To_PCL : Outport
  wires:
  Unit Delay1/1 -> Bus Creator/2  "DistTrvld_m"
  Bus Selector1/2 -> Unit Delay1/1  "<DistTrvld_m>"
  Unit Delay/1 -> Bus Creator/1  "EC_Wh_m"
  Bus Selector1/1 -> Unit Delay/1  "<blndElecEC_Wh_m>"
  Bus Creator/1 -> Series Parallel Hybrid Electric Truck Energy Management System/2(From_PCL_BUS)
  Cd/1 -> 2 DOF Longitudinal Dynamics Model - Force Input/4
  Init_Pos_m/1 -> Series Parallel Hybrid Electric Powertrain Power Loss Model/5(Init_pos_m)
  Bus Selector/1 -> Series Parallel Hybrid Electric Truck Driver and Vehicle Acceleration Dynamics Model - Force Output/2  "<opt_gear>"
  [gear_cmd] -> Bus Creator1/1  "gear_cmd"
  Series Parallel Hybrid Electric Truck Driver and Vehicle Acceleration Dynamics Model - Force Output/1 -> [gear_cmd]
  Series Parallel Hybrid Electric Truck Energy Management System/1(EMC_to_PropSys) -> Series Parallel Hybrid Electric Powertrain Power Loss Model/4(EM_control_bus), Bus Selector/1
  From_PCL/1 -> Bus Creator/3
  2 DOF Longitudinal Dynamics Model - Force Input/4 -> Bus Creator2/2  "F_ar"
  Series Parallel Hybrid Electric Post-Processing/1(To_PCL_BUS) -> To_PCL/1, Bus Selector1/1
  Bus Creator3/1 -> Series Parallel Hybrid Electric Powertrain Power Loss Model/2(Power_data_bus)  "PowerDatBus"
  Bus Selector3/1 -> Series Parallel Hybrid Electric Powertrain Power Loss Model/3(clock)  "<clock>"
  2 DOF Longitudinal Dynamics Model - Force Input/9 -> Bus Creator3/3  "P_cr"
  From_DTIL_BUS/1 -> Bus Selector2/1, Bus Selector3/1
  2 DOF Longitudinal Dynamics Model - Force Input/5 -> Bus Creator2/3  "F_cr"
  V_SPD/1 -> Series Parallel Hybrid Electric Truck Driver and Vehicle Acceleration Dynamics Model - Force Output/3
  2 DOF Longitudinal Dynamics Model - Force Input/2 -> Bus Creator1/4  "vehAccOut"
  Bus Creator1/1 -> Series Parallel Hybrid Electric Powertrain Power Loss Model/1(Motion_data_bus)  "MotionDatBus"
  2 DOF Longitudinal Dynamics Model - Force Input/8 -> Bus Creator3/2  "P_ar"
  2 DOF Longitudinal Dynamics Model - Force Input/10 -> Bus Creator3/4  "P_rr"
  2 DOF Longitudinal Dynamics Model - Force Input/7 -> Bus Creator3/1  "P_prop"
  Bus Creator2/1 -> Terminator/1
  Series Parallel Hybrid Electric Truck Driver and Vehicle Acceleration Dynamics Model - Force Output/3 -> 2 DOF Longitudinal Dynamics Model - Force Input/1  "F_cmd_out"
  2 DOF Longitudinal Dynamics Model - Force Input/1 -> Series Parallel Hybrid Electric Truck Driver and Vehicle Acceleration Dynamics Model - Force Output/1, Bus Creator1/3  "vehSpdOut"
  F_Dist_m/1 -> 2 DOF Longitudinal Dynamics Model - Force Input/3
  2 DOF Longitudinal Dynamics Model - Force Input/6 -> Bus Creator2/4  "F_rr"
  2 DOF Longitudinal Dynamics Model - Force Input/3 -> Bus Creator2/1  "F_prop"
  Bus Selector2/1 -> 2 DOF Longitudinal Dynamics Model - Force Input/2  "<tail_grade_pct>"
  Series Parallel Hybrid Electric Powertrain Power Loss Model/1(PropSys_to_EMC) -> Series Parallel Hybrid Electric Truck Energy Management System/1(PropSys_to_EMC), Series Parallel Hybrid Electric Post-Processing/1(PropSys_to_EMC)
  Series Parallel Hybrid Electric Truck Driver and Vehicle Acceleration Dynamics Model - Force Output/2 -> [gear_ratio]
  [gear_ratio] -> Bus Creator1/2  "gear_ratio"

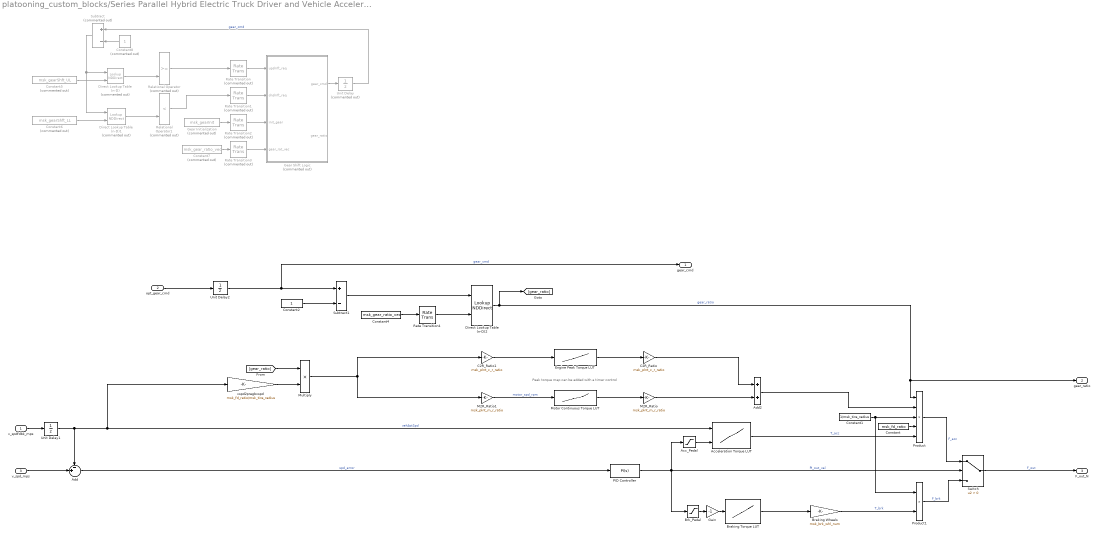
== system platooning_custom_blocks/Series Parallel Hybrid Electric Truck Driver and Vehicle Acceleration Dynamics Model - Force Output ==
  note: Peak torque map can be added with a timer control
  v_spdfdbk_mps : Inport
  opt_gear_cmd : Inport  Port=2
  v_spd_mps : Inport  Port=3
  Acc_Pedal : Saturate  UpperLimit=1  LowerLimit=0
  Acceleration Torque LUT : Lookup_n-D  BreakpointsForDimension1=msk_acc_spdbpt  BreakpointsForDimension2=msk_acc_pdlbpt  Table=msk_acc_trqmap  InternalRulePriority=Speed  RndMeth=Simplest  InputSameDT=on
  Add : Sum  Inputs=-+|
  Add2 : Sum
  Braking Torque LUT : Lookup_n-D  NumberOfTableDimensions=1  BreakpointsForDimension1=msk_brk_pdlbpt  Table=msk_brk_trq * -1  ExtrapMethod=Clip  UseLastTableValue=on  InternalRulePriority=Speed  RndMeth=Simplest  InputSameDT=on
  Braking Wheels : Gain  Gain=msk_brk_whl_num
  Brk_Pedal : Saturate  UpperLimit=0  LowerLimit=-1
  C2R_Ratio : Gain  Gain=msk_plnt_c_r_ratio
  C2R_Ratio1 : Gain  Gain=msk_plnt_c_r_ratio
  Constant : Constant  Value=msk_fd_ratio
  Constant1 : Constant  Value=1/msk_tire_radius
  Constant2 : Constant
  Constant4 : Constant  Value=msk_gear_ratio_vec
  Constant5 : Constant  Commented=on  Value=msk_gearShft_UL
  Constant6 : Constant  Commented=on  Value=msk_gearShft_LL
  Constant7 : Constant  Commented=on  Value=msk_gear_ratio_vec
  Constant8 : Constant  Commented=on
  Direct Lookup Table (n-D) : LookupNDDirect  Commented=on  NumberOfTableDimensions=1  TableIsInput=on
  Direct Lookup Table (n-D)1 : LookupNDDirect  Commented=on  NumberOfTableDimensions=1  TableIsInput=on
  Direct Lookup Table (n-D)2 : LookupNDDirect  NumberOfTableDimensions=1  TableIsInput=on
  Engine Peak Torque LUT : Lookup_n-D  NumberOfTableDimensions=1  BreakpointsForDimension1=msk_eng_spd_bpt  Table=msk_eng_pk_trq  ExtrapMethod=Clip  UseLastTableValue=on  InternalRulePriority=Speed  RndMeth=Simplest  InputSameDT=on
  Gain : Gain  Gain=-1
  Gear Initialization : Constant  Commented=on  Value=msk_gearInit
  Gear Shift Logic : MATLAB Function  Commented=on  TreatAsAtomicUnit=on
  M2R_Ratio : Gain  Gain=msk_plnt_m_r_ratio
  M2R_Ratio1 : Gain  Gain=msk_plnt_m_r_ratio
  Motor Continuous Torque LUT : Lookup_n-D  NumberOfTableDimensions=1  BreakpointsForDimension1=msk_spd_bpt  Table=msk_mtr_cont_trq  ExtrapMethod=Clip  UseLastTableValue=on  InternalRulePriority=Speed  RndMeth=Simplest  InputSameDT=on
  Multiply : Product
  PID Controller : simulink/Continuous/PID Controller  Controller=PI  Form=Parallel  TimeDomain=Continuous-time  SampleTime=-1  IntegratorMethod=Forward Euler  FilterMethod=Forward Euler  ControllerParametersSource=internal  P=msk_Kp  I=msk_Ki  D=0  UseFilter=on  N=100  TunerSelectOption=Transfer Function Based (PID Tuner App)  InitialConditionSource=internal  InitialConditionForIntegrator=0  InitialConditionForFilter=0  DifferentiatorICPrevScaledInput=0  ExternalReset=none  TrackingMode=off  Kt=1  LimitOutput=on  UpperSaturationLimit=1  LowerSaturationLimit=-1  LinearizeAsGain=on  AntiWindupMode=clamping  Kb=1  POutMin=[]  POutMax=[]  IOutMin=[]  IOutMax=[]  DOutMin=[]  DOutMax=[]  NOutMin=[]  NOutMax=[]  SumOutMin=[]  SumOutMax=[]  SaturationOutMin=[]  SaturationOutMax=[]  PParamMin=[]  PParamMax=[]  IParamMin=[]  IParamMax=[]  DParamMin=[]  DParamMax=[]  NParamMin=[]  NParamMax=[]  KbParamMin=[]  KbParamMax=[]  KtParamMin=[]  KtParamMax=[]  KbOutMin=[]  KbOutMax=[]  KtOutMin=[]  KtOutMax=[]  IntegratorOutMin=[]  IntegratorOutMax=[]  FilterOutMin=[]  FilterOutMax=[]  SumI1OutMin=[]  SumI1OutMax=[]  SumI2OutMin=[]  SumI2OutMax=[]  SumI3OutMin=[]  SumI3OutMax=[]  SumI4OutMin=[]  SumI4OutMax=[]  SumDOutMin=[]  SumDOutMax=[]  DifferentiatorOutMin=[]  DifferentiatorOutMax=[]  FilterDiffOutCoefMin=[]  FilterDiffOutCoefMax=[]  ReciprocalOutMin=[]  ReciprocalOutMax=[]  SumDenOutMin=[]  SumDenOutMax=[]  SumNumOutMin=[]  SumNumOutMax=[]  DivideOutMin=[]  DivideOutMax=[]  IntegratorContinuousStateAttributes=''  IntegratorStateMustResolveToSignalObject=off  IntegratorRTWStateStorageClass=Auto  FilterContinuousStateAttributes=''  FilterStateMustResolveToSignalObject=off  FilterRTWStateStorageClass=Auto  ParallelPVariant=InternalParameters  IdealPVariant=Disabled  IVariant=InternalParameters  DVariant=Disabled  IntegratorVariant=Continuous  SatVariant=Enabled  AWVariant=ContClampingParallel  PCopyVariant=Disabled  TRVariant=Disabled  FdbkBlocksVariant=Forward  IdealPFdbkVariant=Disabled  SatFdbkVariant=Disabled  DerivativeFilterVariant=Disabled  NVariant=Disabled  NCopyVariant=Disabled_SignalSpec  FilterICVariant=Disabled  IntegratorICVariant=InternalICs  ExternalResetVariant=Disabled  TRSumVariant=Passthrough  SumFdbkVariant=Disabled  SumVariant=Sum_PI
  Product : Product  Inputs=5
  Product1 : Product
  Rate Transition{,1..3} (4 alike) : RateTransition  Commented=on  OutPortSampleTime=msk_t_step
  Rate Transition4 : RateTransition  OutPortSampleTime=msk_t_step
  Relational Operator : RelationalOperator  Commented=on  OutDataTypeStr=boolean  RndMeth=Simplest
  Relational Operator1 : RelationalOperator  Commented=on  Operator=<  OutDataTypeStr=boolean  RndMeth=Simplest
  Subtract : Sum  Commented=on  Inputs=+-
  Subtract1 : Sum  Inputs=+-
  Switch : Switch  Criteria=u2 > Threshold
  Unit Delay : UnitDelay  Commented=on  SampleTime=-1
  Unit Delay1 : UnitDelay  SampleTime=-1
  Unit Delay2 : UnitDelay  InitialCondition=msk_gearInit  SampleTime=-1
  vspd2pregbxspd : Gain  Gain=msk_fd_ratio/msk_tire_radius
  gear_cmd : Outport
  gear_ratio : Outport  Port=2
  F_out_N : Outport  Port=3
  wires:
  Gain/1 -> Braking Torque LUT/1
  Brk_Pedal/1 -> Gain/1
  Multiply/1 -> C2R_Ratio1/1, M2R_Ratio1/1
  [gear_ratio] -> Multiply/1
  vspd2pregbxspd/1 -> Multiply/2
  C2R_Ratio1/1 -> Engine Peak Torque LUT/1
  M2R_Ratio/1 -> Add2/2
  C2R_Ratio/1 -> Add2/1
  Engine Peak Torque LUT/1 -> C2R_Ratio/1
  Add2/1 -> Product/2
  Relational Operator/1 -> Rate Transition/1
  Rate Transition/1 -> Gear Shift Logic/1(upshift_req)
  Constant7/1 -> Rate Transition3/1
  Gear Shift Logic/1(gear_cmd) -> Unit Delay/1
  Rate Transition1/1 -> Gear Shift Logic/2(dnshift_req)
  Subtract/1 -> Direct Lookup Table (n-D)/1, Direct Lookup Table (n-D)1/1
  Direct Lookup Table (n-D)/1 -> Relational Operator/2
  Relational Operator1/1 -> Rate Transition1/1
  Constant8/1 -> Subtract/2
  Gear Initialization/1 -> Rate Transition2/1
  Constant6/1 -> Direct Lookup Table (n-D)1/2
  Direct Lookup Table (n-D)1/1 -> Relational Operator1/2
  Rate Transition2/1 -> Gear Shift Logic/3(init_gear)
  Direct Lookup Table (n-D)2/1 -> gear_ratio/1, Product/1, [gear_ratio]  "gear_ratio"
  Unit Delay/1 -> Subtract/1  "gear_cmd"
  Rate Transition3/1 -> Gear Shift Logic/4(gear_rat_vec)
  Constant5/1 -> Direct Lookup Table (n-D)/2
  Unit Delay1/1 -> Add/1, vspd2pregbxspd/1, Acceleration Torque LUT/1  "vehActSpd"
  Switch/1 -> F_out_N/1  "F_out"
  Braking Wheels/1 -> Product1/2  "T_brk"
  Acceleration Torque LUT/1 -> Product/5  "T_acc"
  Braking Torque LUT/1 -> Braking Wheels/1
  PID Controller/1 -> Switch/2, Acc_Pedal/1, Brk_Pedal/1  "PI_out_val"
  v_spdfdbk_mps/1 -> Unit Delay1/1
  v_spd_mps/1 -> Add/2
  Product1/1 -> Switch/3  "F_brk"
  Product/1 -> Switch/1  "F_acc"
  Add/1 -> PID Controller/1  "spd_error"
  Acc_Pedal/1 -> Acceleration Torque LUT/2
  Constant/1 -> Product/4
  Constant1/1 -> Product/3, Product1/1
  Motor Continuous Torque LUT/1 -> M2R_Ratio/1
  M2R_Ratio1/1 -> Motor Continuous Torque LUT/1  "motor_spd_rpm"
  Unit Delay2/1 -> gear_cmd/1, Subtract1/1  "gear_cmd"
  Constant2/1 -> Subtract1/2
  Subtract1/1 -> Direct Lookup Table (n-D)2/1
  Rate Transition4/1 -> Direct Lookup Table (n-D)2/2
  opt_gear_cmd/1 -> Unit Delay2/1
  Constant4/1 -> Rate Transition4/1

== system platooning_custom_blocks/Tail Truck Powertrain Variant Subsystem ==
  note: 1) Add Subsystem or Model blocks as valid variant choices.
      | 2) You cannot connect blocks at this level. At simulation, connectivity is automatically
      | determined, based on the active variant and port name matching.
  From_DTIL_BUS : Inport
  V_SPD : Inport  Port=2
  F_Dist_m : Inport  Port=3
  Cd : Inport  Port=4
  From_PCL : Inport  Port=5
  Init_Pos_m : Inport  Port=6
  Battery Electric Truck : $bdroot/Battery Electric Truck  SystemSampleTime=-1  VariantControl=TT.Type == 3
  Conventional Truck : $bdroot/Conventional Truck  SystemSampleTime=-1  VariantControl=TT.Type == 1
  Series Parallel Hybrid Electric Truck : $bdroot/Series Parallel Hybrid Electric Truck  SystemSampleTime=-1  VariantControl=TT.Type == 2
  To_PCL : Outport

== system platooning_custom_blocks/V2V Communication Block ==
  sig_in : Inport
  T_DELAY_S : Inport  Port=2
  Constant1 : Constant  Value=msk_t_step_s
  Constant2 : Constant  Value=msk_snr_value
  V2V Communication Delay Funtion : MATLAB Function  TreatAsAtomicUnit=on
  sig_out : Outport
  wires:
  sig_in/1 -> V2V Communication Delay Funtion/1(sig_in)
  Constant1/1 -> V2V Communication Delay Funtion/3(T_STEP)
  V2V Communication Delay Funtion/1(sig_out) -> sig_out/1  "sig_out"
  T_DELAY_S/1 -> V2V Communication Delay Funtion/2(T_DELAY)
  Constant2/1 -> V2V Communication Delay Funtion/4(SNR_VALUE)

== system platooning_custom_blocks/Battery Electric Truck/Battery Electric Post-Processing ==
  PropSys_to_EMC : Inport
  Battery Energy Max : Constant  Value=msk_batt_Ns * msk_batt_Np * msk_batt_Nmod * msk_cell_Vnom * msk_cell_Q_Ah
  Blending Function : Subsystem
  Bus Creator : BusCreator  Inputs=3
  Bus Creator1 : BusCreator  Inputs=8
  Bus Creator2 : BusCreator  Inputs=3
  Bus Creator3 : BusCreator  Inputs=3
  Bus Selector : BusSelector  OutputSignals=Batt_SOC_frac,DistTrvld_m,Init_Pos_m,act_VehSpd_mps,Batt_Load_Voltage,Batt_Current_Ampere,Batt_EPO_Flag,P_elec_dem_W
  Constant : Constant  Value=msk_batt_soc_init
  Constant1 : Constant  Value=NaN
  Constant2 : Constant  Value=NaN
  Constant3 : Constant  Value=NaN
  Distance to Empty Calculator : Subsystem
  Divide : Product  Inputs=*/
  Product : Product
  Rate Transition : RateTransition  OutPortSampleTime=sim_t_step
  Rate Transition1 : RateTransition  OutPortSampleTime=sim_t_step
  Short Term Averaging Function : MATLAB Function  TreatAsAtomicUnit=on
  Short term average distance window - meters : Constant  Value=msk_distwin
  Subtract : Sum  Inputs=+-
  Subtract1 : Sum  Inputs=+-
  To_PCL_BUS : Outport
  wires:
  Bus Selector/3 -> Subtract1/2  "<Init_Pos_m>"
  Bus Selector/2 -> Subtract1/1, Bus Creator1/3  "<DistTrvld_m>"
  Bus Creator3/1 -> Bus Creator2/1  "FC_BUS"
  Constant3/1 -> Bus Creator3/1  "runAvgFuelEC_Wh_m"
  Constant2/1 -> Bus Creator3/2  "blndFuelEC_Wh_m"
  Constant1/1 -> Bus Creator3/3  "stAvgFuelEC_Wh_m"
  Bus Selector/8 -> Bus Creator1/8  "<P_elec_dem_W>"
  Bus Selector/7 -> Bus Creator1/7  "<Batt_EPO_Flag>"
  Bus Selector/6 -> Bus Creator1/6  "<Batt_Current_Ampere>"
  Bus Selector/5 -> Bus Creator1/5  "<Batt_Load_Voltage>"
  Distance to Empty Calculator/1(estDTE_km) -> Bus Creator1/1  "estDTE_km"
  Rate Transition1/1 -> Distance to Empty Calculator/2(battSOC_frac), Blending Function/2(<Batt_SOC_frac>), Short Term Averaging Function/1(Batt_SOC_frac)
  Rate Transition/1 -> Divide/2
  PropSys_to_EMC/1 -> Bus Selector/1
  Bus Selector/1 -> Subtract/2, Bus Creator1/2, Rate Transition1/1  "<Batt_SOC_frac>"
  Constant/1 -> Subtract/1
  Subtract/1 -> Product/2
  Product/1 -> Divide/1
  Subtract1/1 -> Rate Transition/1, Short Term Averaging Function/2(Dist_Travelled)  "DistTrvld_m"
  Divide/1 -> Blending Function/1(runAvgElecEC_Wh_m), Bus Creator/1  "runAvgElecEC_Wh_m"
  Short term average distance window - meters/1 -> Short Term Averaging Function/4(Dist_Window)
  Battery Energy Max/1 -> Short Term Averaging Function/3(Batt_Max_Energy), Product/1
  Short Term Averaging Function/1(STAvg_Wh_m) -> Blending Function/3(stAvgElecEC_Wh_m), Bus Creator/3  "stAvgElecEC_Wh_m"
  Blending Function/1(blndElecEC_Wh_m) -> Bus Creator/2, Distance to Empty Calculator/1(blndEC_Wh_m)  "blndElecEC_Wh_m"
  Bus Creator/1 -> Bus Creator2/2  "EC_BUS"
  Bus Selector/4 -> Bus Creator1/4  "<act_VehSpd_mps>"
  Bus Creator1/1 -> Bus Creator2/3  "State_BUS"
  Bus Creator2/1 -> To_PCL_BUS/1
